simulink model "singleVehicleModel"  (R2021a)
settings: Solver=VariableStepAuto  StartTime=0.0  StopTime=inf  RelTol=1e-3
values from neighbouring files (symbols this model uses):
  curvature = (dx.*d2y - dy.*d2x) ./(dx.^2+dy.^2).^(3/2)    [RRTstar_planner.m]
  dist_ref = (linspace(0,dist(end,1),50))'    [RRTstar_planner.m]
  theta_0 = theta_ref2(1,1)    [RRTstar_planner.m]
  theta_ref2 = ppval(theta_cs,dist_ref)    [RRTstar_planner.m]
  x_0 = x_ref2(1,1)    [RRTstar_planner.m]
  x_ref2 = ppval(x_cs,dist_ref)    [RRTstar_planner.m]
  y_0 = y_ref2(1,1)    [RRTstar_planner.m]
  y_ref2 = ppval(y_cs,dist_ref)    [RRTstar_planner.m]
libraries: simulink_extras x3, drivingvehiclecontroller x1, autolibshared x1, simulink x1
settings Model: Creator=vasud  LastModifiedBy=vasud

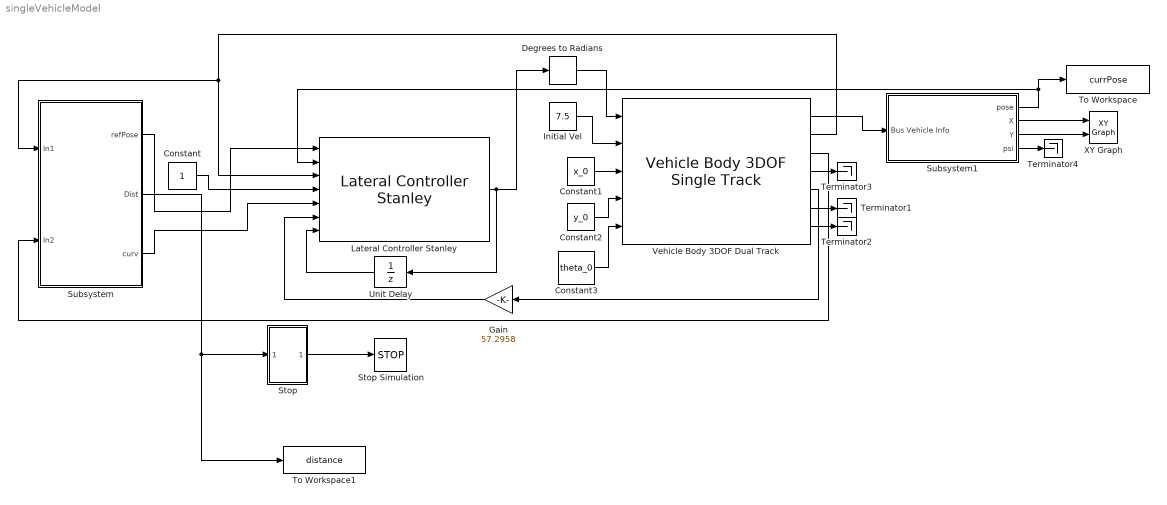
== system singleVehicleModel ==
  Constant : Constant
  Constant1 : Constant  Value=x_0
  Constant2 : Constant  Value=y_0
  Constant3 : Constant  Value=theta_0
  Degrees to Radians : simulink_extras/Transformations/Degrees to Radians
  Gain : Gain  Gain=57.2958
  Initial Vel : Constant  Value=7.5
  Lateral Controller Stanley : drivingvehiclecontroller/Lateral Controller Stanley  ModelType=Dynamic bicycle model  PositionGainF=4.3  PositionGainR=1  YawRateGain=0.8  DelayGain=0.81  VehicleMass=1575  Lf=1.2  Lr=1.6  TireStiffness=19000  Wheelbase=2.8  MaxSteeringAngle=40
      settings: SourceProductBaseCode=DR
  Stop : Subsystem
  Stop Simulation : Stop
  Subsystem : Subsystem
  Subsystem1 : Subsystem
  Terminator{1..4} (4 alike) : Terminator
  To Workspace : ToWorkspace  VariableName=currPose  SaveFormat=Timeseries  SampleTime=-1
  To Workspace1 : ToWorkspace  VariableName=distance  SaveFormat=Timeseries  SampleTime=-1
  Unit Delay : UnitDelay  SampleTime=-1  HasFrameUpgradeWarning=on
  Vehicle Body 3DOF Dual Track : autolibshared/Vehicle Body 3DOF Single Track  trackMode=Dual  inputMode=External longitudinal velocity  frontSteerMode=on  rearSteerMode=off  windMode=off  muMode=off  extFMode=off  extMMode=off  htchFMode=off  htchMMode=off  extXo=on  extpsio=on  extxdoto=off  extro=off  extYo=on  extTamb=off  extydoto=off  aMode=2  NF=2  NR=2  m=2000  a=1.4  b=1.6  h=0.35  dh=1  hh=0.2  X_o=0  xdot_o=0  CalphaMode=off  sigmaMode=on  d=0  hl=0  w=[1.4,1.4]  Cy_f=12e3  Cy_r=11e3  sigma_f=.1  sigma_r=.1  alpha_f_brk=[-.1 .1]  Cy_f_data=[-9e3 9e3]  alpha_r_brk=[-.1 .1]  Cy_r_data=[-9e3 9e3]  Y_o=0  ydot_o=0  Izz=4000  psi_o=0  r_o=0  Af=2  Cd=.3  Cl=.1  Cpm=.1  beta_w=[0:0.01:0.3]  Cs=[0:0.03:0.9]  Cym=[0:0.01:0.3]  Pabs=101325  Tair=273  g=9.81  mu=1  xdot_tol=.01  Fznom=5000  Fxtire_sat=7e4  Fytire_sat=7e4  longOff=0  latOff=0  vertOff=0  wrapAng=off
      settings: SourceProductBaseCode=PW,DR,MT,UV,VE
  XY Graph : simulink/Sinks/XY Graph  xmin=0  xmax=x_size  ymin=0  ymax=y_size  st=-1
  wires:
  Constant/1 -> Lateral Controller Stanley/4
  Vehicle Body 3DOF Dual Track/2 -> Lateral Controller Stanley/3, Subsystem/1(In1)
  Vehicle Body 3DOF Dual Track/3 -> Subsystem/2(In2)
  Subsystem/1(refPose) -> Lateral Controller Stanley/1
  Lateral Controller Stanley/1 -> Degrees to Radians/1, Unit Delay/1
  Degrees to Radians/1 -> Vehicle Body 3DOF Dual Track/1
  Initial Vel/1 -> Vehicle Body 3DOF Dual Track/2
  Vehicle Body 3DOF Dual Track/5 -> Gain/1
  Vehicle Body 3DOF Dual Track/6 -> Terminator1/1
  Vehicle Body 3DOF Dual Track/7 -> Terminator2/1
  Vehicle Body 3DOF Dual Track/1 -> Subsystem1/1(Bus Vehicle Info)
  Subsystem1/1(pose) -> To Workspace/1, Lateral Controller Stanley/2
  Vehicle Body 3DOF Dual Track/4 -> Terminator3/1
  Stop/1(Stop) -> Stop Simulation/1
  Constant1/1 -> Vehicle Body 3DOF Dual Track/3
  Constant2/1 -> Vehicle Body 3DOF Dual Track/4
  Constant3/1 -> Vehicle Body 3DOF Dual Track/5
  Subsystem/2(Dist) -> To Workspace1/1, Stop/1(Dist)
  Subsystem1/2(X) -> XY Graph/1
  Subsystem1/3(Y) -> XY Graph/2
  Subsystem1/4(psi) -> Terminator4/1
  Unit Delay/1 -> Lateral Controller Stanley/7
  Subsystem/3(curv) -> Lateral Controller Stanley/5
  Gain/1 -> Lateral Controller Stanley/6

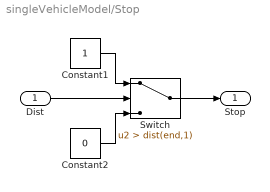
== system singleVehicleModel/Stop ==
  Dist : Inport
  Constant1 : Constant
  Constant2 : Constant  Value=0
  Switch : Switch  Criteria=u2 > Threshold  Threshold=dist(end,1)
  Stop : Outport
  wires:
  Constant2/1 -> Switch/3
  Constant1/1 -> Switch/1
  Switch/1 -> Stop/1
  Dist/1 -> Switch/2

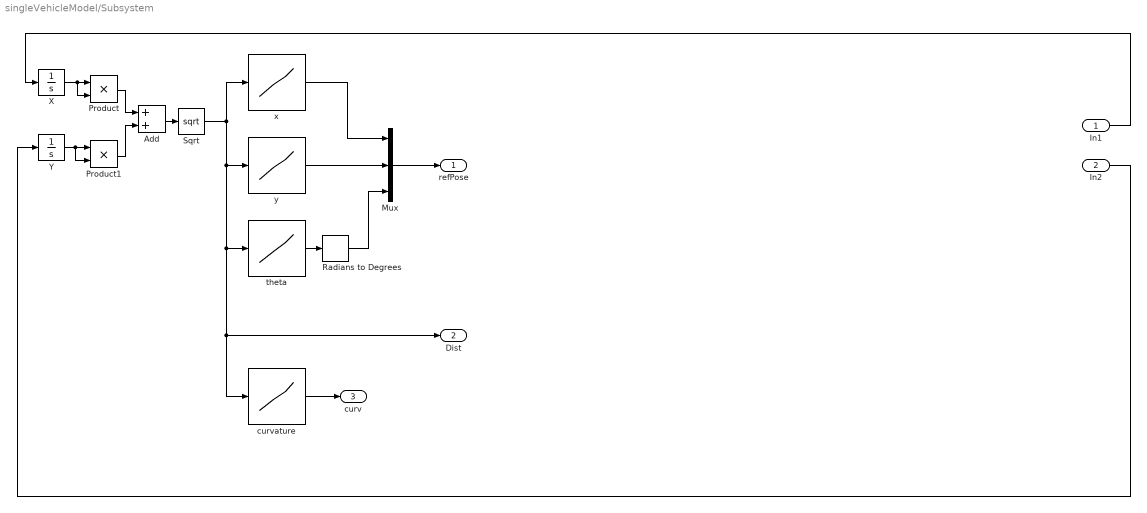
== system singleVehicleModel/Subsystem ==
  In1 : Inport
  In2 : Inport  Port=2
  Add : Sum
  Mux : Mux  Inputs=3
  Product : Product
  Product1 : Product
  Radians to Degrees : simulink_extras/Transformations/Radians to Degrees
  Sqrt : Sqrt  SaturateOnIntegerOverflow=on
  X : Integrator
  Y : Integrator
  curvature : Lookup_n-D  NumberOfTableDimensions=1  BreakpointsForDimension1=dist_ref  BreakpointsForDimension3=[5, 7]  Table=curvature  InternalRulePriority=Speed  RndMeth=Simplest  InputSameDT=on
  theta : Lookup_n-D  NumberOfTableDimensions=1  BreakpointsForDimension1=dist_ref  BreakpointsForDimension3=[5, 7]  Table=theta_ref2  InternalRulePriority=Speed  RndMeth=Simplest  InputSameDT=on
  x : Lookup_n-D  NumberOfTableDimensions=1  BreakpointsForDimension1=dist_ref  BreakpointsForDimension3=[5, 7]  Table=x_ref2  InternalRulePriority=Speed  RndMeth=Simplest  InputSameDT=on
  y : Lookup_n-D  NumberOfTableDimensions=1  BreakpointsForDimension1=dist_ref  BreakpointsForDimension3=[5, 7]  Table=y_ref2  InternalRulePriority=Speed  RndMeth=Simplest  InputSameDT=on
  refPose : Outport
  Dist : Outport  Port=2
  curv : Outport  Port=3
  wires:
  x/1 -> Mux/1
  Radians to Degrees/1 -> Mux/3
  y/1 -> Mux/2
  theta/1 -> Radians to Degrees/1
  Mux/1 -> refPose/1
  In1/1 -> X/1
  curvature/1 -> curv/1
  In2/1 -> Y/1
  X/1 -> Product/2, Product/1
  Y/1 -> Product1/2, Product1/1
  Product/1 -> Add/1
  Product1/1 -> Add/2
  Add/1 -> Sqrt/1
  Sqrt/1 -> x/1, Dist/1, curvature/1, theta/1, y/1

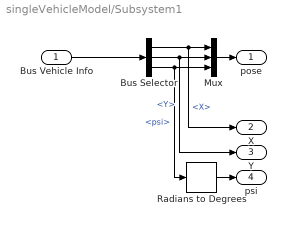
== system singleVehicleModel/Subsystem1 ==
  Bus Vehicle Info : Inport
  Bus Selector : BusSelector  OutputSignals=InertFrm.Cg.Disp.X,InertFrm.Cg.Disp.Y,InertFrm.Cg.Ang.psi
  Mux : Mux  Inputs=3
  Radians to Degrees : simulink_extras/Transformations/Radians to Degrees
  pose : Outport
  X : Outport  Port=2
  Y : Outport  Port=3
  psi : Outport  Port=4
  wires:
  Bus Selector/2 -> Y/1, Mux/2  "<Y>"
  Bus Vehicle Info/1 -> Bus Selector/1
  Bus Selector/3 -> Radians to Degrees/1, Mux/3  "<psi>"
  Bus Selector/1 -> X/1, Mux/1  "<X>"
  Mux/1 -> pose/1
  Radians to Degrees/1 -> psi/1
